simulink model "LQR_Model"  (R2015b)
settings: Solver=VariableStepAuto  StartTime=0.0  StopTime=100  RelTol=1e-3
values from neighbouring files (symbols this model uses):
  K = [0.133180472867 -0.360593186384 0.174341644763]    [matlab.mat]
  LQR = [-0.566321569976 0.00826847649943 0 9.99988971029 9.8593256098 -0.500173757981 0 79.9164329174 -0.0826847649943 9.99988971029 0 174.999862655 ... (16 elements, 4x4)]    [matlab.mat]
undefined symbols (not defined in the file or in its folder): sys_d
settings Model: Creator=Jcama  LastModifiedBy=Jcama

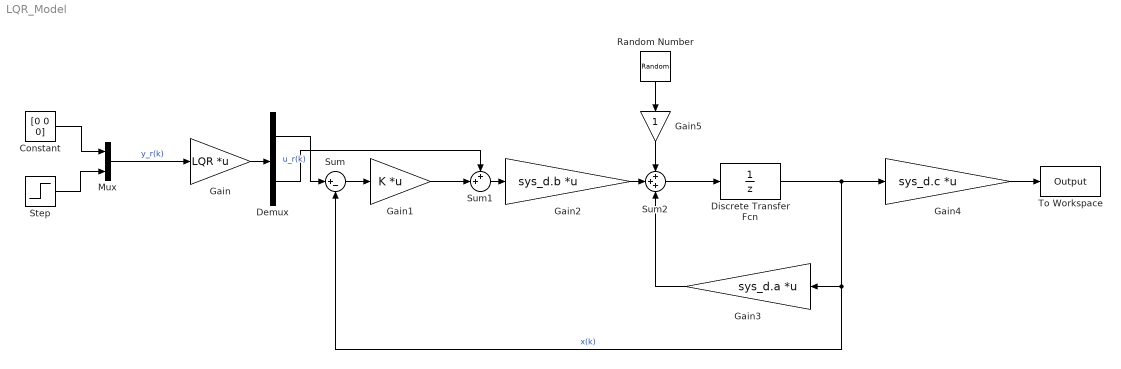
== system LQR_Model ==
  Constant : Constant  Value=[0 0 0]
  Demux : Demux  Outputs=[3 1]
  Discrete Transfer Fcn : DiscreteTransferFcn  Denominator=[1 0]
  Gain : Gain  Gain=LQR  Multiplication=Matrix(K*u)
  Gain1 : Gain  Gain=K  Multiplication=Matrix(K*u)
  Gain2 : Gain  Gain=sys_d.b  Multiplication=Matrix(K*u)
  Gain3 : Gain  Gain=sys_d.a  Multiplication=Matrix(K*u)
  Gain4 : Gain  Gain=sys_d.c  Multiplication=Matrix(K*u)
  Gain5 : Gain
  Mux : Mux  Inputs=2
  Random Number : RandomNumber  Variance=0.6  SampleTime=0.1
  Step : Step  After=80  SampleTime=0.1
  Sum : Sum  Inputs=|+-
  Sum1 : Sum  Inputs=++|
  Sum2 : Sum  Inputs=+++
  To Workspace : ToWorkspace  VariableName=Output  SaveFormat=Timeseries  SampleTime=0.1
  wires:
  Gain/1 -> Demux/1
  Sum/1 -> Gain1/1
  Gain1/1 -> Sum1/2
  Sum1/1 -> Gain2/1
  Sum2/1 -> Discrete Transfer Fcn/1
  Discrete Transfer Fcn/1 -> Gain4/1, Sum/2, Gain3/1  "x(k)"
  Gain4/1 -> To Workspace/1
  Gain2/1 -> Sum2/2
  Gain3/1 -> Sum2/3
  Gain5/1 -> Sum2/1
  Random Number/1 -> Gain5/1
  Mux/1 -> Gain/1  "y_r(k)"
  Demux/2 -> Sum1/1
  Demux/1 -> Sum/1  "u_r(k)"
  Constant/1 -> Mux/1
  Step/1 -> Mux/2
